simulink model "dfl_model"  (R2022b)
settings: Solver=VariableStepAuto  StartTime=0.0  StopTime=15.0  FixedStep=0.05  RelTol=1e-3
InitFcn:
  | port = 19999;
  | InitSim;
values from neighbouring files (symbols this model uses):
  p = [m, g, I_x, I_y, I_z, c0, c1, c2, c3]'    [dfl_params.m]
  state0 = [x0 y0 z0 v_x0 v_y0 v_z0 phi0 th0 psi0 w_x0 w_y0 w_z0]'    [dfl_params.m]
libraries: VrepLib x1, PosLib x1
settings Model: Creator=dorec  LastModifiedBy=dorec
settings DebuggingCC: SignalInfNanChecking=error

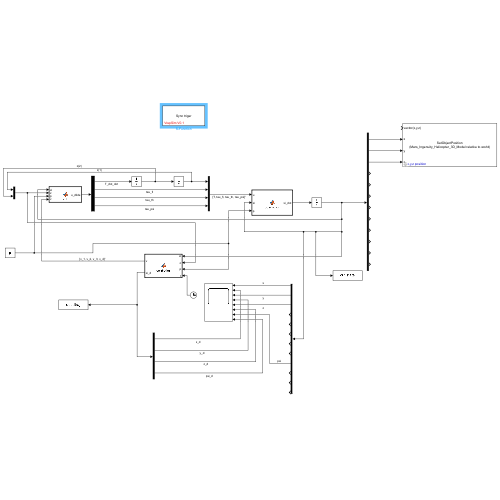
[thumbnail: Simulink's stored preview of the top-level diagram]
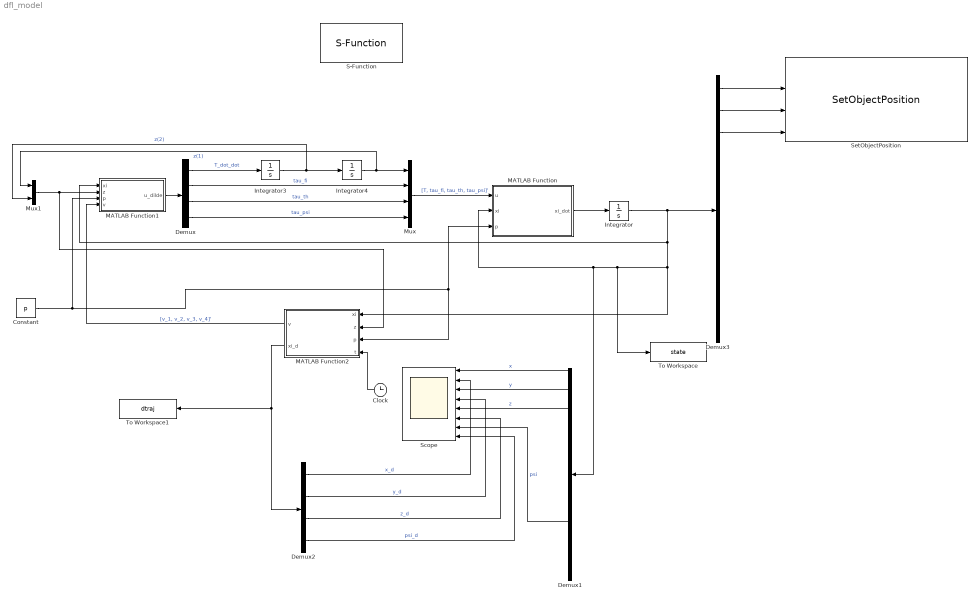
== system dfl_model ==
  Clock : Clock
  Constant : Constant  Value=p
  Demux : Demux
  Demux1 : Demux  Outputs=12
  Demux2 : Demux
  Demux3 : Demux  Outputs=12
  Integrator : Integrator  InitialCondition=state0
  Integrator3 : Integrator
  Integrator4 : Integrator  InitialCondition=1
  MATLAB Function : MATLAB Function  TreatAsAtomicUnit=on
  MATLAB Function1 : MATLAB Function  TreatAsAtomicUnit=on
  MATLAB Function2 : MATLAB Function  TreatAsAtomicUnit=on
  Mux : Mux
  Mux1 : Mux  Inputs=2
  S-Function : VrepLib/S-Function  SFunctionModules=''
      settings: SourceProductName=VrepLib
  Scope : Scope  NumInputPorts=8
  SetObjectPosition : PosLib/SetObjectPosition  object_name='Mars_Ingenuity_Helicopter_3D_Model'  relative_object_name='world'  isUseVector=off
  To Workspace : ToWorkspace  VariableName=state  SaveFormat=Timeseries  SampleTime=-1
  To Workspace1 : ToWorkspace  VariableName=dtraj  SaveFormat=Timeseries  SampleTime=-1
  wires:
  MATLAB Function/1(xi_dot) -> Integrator/1
  Integrator/1 -> MATLAB Function1/1(xi), To Workspace/1, Demux1/1, MATLAB Function/2(xi), MATLAB Function2/1(xi), Demux3/1
  Mux/1 -> MATLAB Function/1(u)  "[T, tau_fi, tau_th, tau_psi]'"
  MATLAB Function1/1(u_dilde) -> Demux/1
  Demux/1 -> Integrator3/1  "T_dot_dot"
  MATLAB Function2/1(v) -> MATLAB Function1/4(v)  "[v_1, v_2, v_3, v_4]'"
  Demux/3 -> Mux/3  "tau_th"
  Demux/2 -> Mux/2  "tau_fi"
  Mux1/1 -> MATLAB Function2/2(z), MATLAB Function1/2(z)
  Constant/1 -> MATLAB Function1/3(p), MATLAB Function/3(p), MATLAB Function2/3(p)
  Clock/1 -> MATLAB Function2/4(t)
  Integrator3/1 -> Mux1/2, Integrator4/1  "z(2)"
  Integrator4/1 -> Mux1/1, Mux/1  "z(1)"
  Demux/4 -> Mux/4  "tau_psi"
  Demux1/1 -> Scope/1  "x"
  Demux1/2 -> Scope/3  "y"
  Demux1/3 -> Scope/5  "z"
  MATLAB Function2/2(xi_d) -> To Workspace1/1, Demux2/1
  Demux2/1 -> Scope/2  "x_d"
  Demux2/2 -> Scope/4  "y_d"
  Demux2/3 -> Scope/6  "z_d"
  Demux2/4 -> Scope/8  "psi_d"
  Demux1/9 -> Scope/7  "psi"
  Demux3/1 -> SetObjectPosition/2
  Demux3/2 -> SetObjectPosition/3
  Demux3/3 -> SetObjectPosition/4

== matlab function dfl_model/MATLAB Function1 ==
  data: xi input size=12; z input size=2; p input size=9; u_dilde output size=4; v input size=4
function u_dilde = dfl(xi, z, p, v)

% x = xi(1);
% y = xi(2);
% z = xi(3);
% v_x = xi(4);
% v_y = xi(5);
% v_z = xi(6);
fi = xi(7);
th = xi(8);
psi = xi(9);
w_x = xi(10);
w_y = xi(11);
w_z = xi(12);

m = p(1);
% g = p(2);
I_x = p(3);
I_y = p(4);
I_z = p(5);

T = z(1);
T_dot = z(2);

J_1 = [-(m*(sin(fi)*sin(psi) + cos(fi)*cos(psi)*sin(th)))/(2*cos(fi)^2*cos(psi)^2 - 2*cos(psi)^2 + 2*cos(psi)^2*cos(th)^2 - 2*cos(fi)^2*cos(psi)^2*cos(th)^2 + 2*cos(fi)*cos(psi)*sin(fi)*sin(psi)*sin(th) + 1), ...
    -(m*(cos(psi)*sin(fi) - 2*cos(psi)*cos(th)^2*sin(fi) + cos(fi)*sin(psi)*sin(th)))/(2*cos(fi)^2*cos(psi)^2 - 2*cos(psi)^2 + 2*cos(psi)^2*cos(th)^2 - 2*cos(fi)^2*cos(psi)^2*cos(th)^2 + 2*cos(fi)*cos(psi)*sin(fi)*sin(psi)*sin(th) + 1), ...
    -(m*cos(th)*(cos(fi) + 2*cos(psi)*sin(fi)*sin(psi)*sin(th)))/(2*cos(fi)^2*cos(psi)^2 - 2*cos(psi)^2 + 2*cos(psi)^2*cos(th)^2 - 2*cos(fi)^2*cos(psi)^2*cos(th)^2 + 2*cos(fi)*cos(psi)*sin(fi)*sin(psi)*sin(th) + 1), ...
    (2*T*cos(psi)*(cos(th)^2 - 1)*(sin(psi) - cos(fi)^2*sin(psi) + cos(fi)*cos(psi)*sin(fi)*sin(th)))/(2*cos(fi)^2*cos(psi)^2 - 2*cos(psi)^2 + 2*cos(psi)^2*cos(th)^2 - 2*cos(fi)^2*cos(psi)^2*cos(th)^2 + 2*cos(fi)*cos(psi)*sin(fi)*sin(psi)*sin(th) + 1)];
J_2 = [-(I_x*m*(cos(fi)*sin(psi) - cos(psi)*sin(fi)*sin(th)))/(T*(2*cos(fi)^2*cos(psi)^2 - 2*cos(psi)^2 + 2*cos(psi)^2*cos(th)^2 - 2*cos(fi)^2*cos(psi)^2*cos(th)^2 + 2*cos(fi)*cos(psi)*sin(fi)*sin(psi)*sin(th) + 1)), ...
    (I_x*m*(cos(fi)*cos(psi) + sin(fi)*sin(psi)*sin(th)))/(T*(2*cos(fi)^2*cos(psi)^2 - 2*cos(psi)^2 + 2*cos(psi)^2*cos(th)^2 - 2*cos(fi)^2*cos(psi)^2*cos(th)^2 + 2*cos(fi)*cos(psi)*sin(fi)*sin(psi)*sin(th) + 1)), ...
    (I_x*m*cos(th)*sin(fi))/(T*(2*cos(fi)^2*cos(psi)^2 - 2*cos(psi)^2 + 2*cos(psi)^2*cos(th)^2 - 2*cos(fi)^2*cos(psi)^2*cos(th)^2 + 2*cos(fi)*cos(psi)*sin(fi)*sin(psi)*sin(th) + 1)), ...
    (I_x*sin(th))/(2*cos(fi)^2*cos(psi)^2 - 2*cos(psi)^2 + 2*cos(psi)^2*cos(th)^2 - 2*cos(fi)^2*cos(psi)^2*cos(th)^2 + 2*cos(fi)*cos(psi)*sin(fi)*sin(psi)*sin(th) + 1)];
J_3 = [-(I_y*m*cos(psi)*cos(th))/(T*cos(fi)*(2*cos(fi)^2*cos(psi)^2 - 2*cos(psi)^2 + 2*cos(psi)^2*cos(th)^2 - 2*cos(fi)^2*cos(psi)^2*cos(th)^2 + 2*cos(fi)*cos(psi)*sin(fi)*sin(psi)*sin(th) + 1)), ...
    -(I_y*m*cos(th)*(sin(psi) + 2*cos(fi)*cos(psi)*sin(fi)*sin(th)))/(T*cos(fi)*(2*cos(fi)^2*cos(psi)^2 - 2*cos(psi)^2 + 2*cos(psi)^2*cos(th)^2 - 2*cos(fi)^2*cos(psi)^2*cos(th)^2 + 2*cos(fi)*cos(psi)*sin(fi)*sin(psi)*sin(th) + 1)), ...
    (I_y*m*(sin(th) - 2*cos(psi)^2*sin(th) + 2*cos(fi)^2*cos(psi)^2*sin(th) + 2*cos(fi)*cos(psi)*sin(fi)*sin(psi) - 2*cos(fi)*cos(psi)*cos(th)^2*sin(fi)*sin(psi)))/(T*cos(fi)*(2*cos(fi)^2*cos(psi)^2 - 2*cos(psi)^2 + 2*cos(psi)^2*cos(th)^2 - 2*cos(fi)^2*cos(psi)^2*cos(th)^2 + 2*cos(fi)*cos(psi)*sin(fi)*sin(psi)*sin(th) + 1)), ...
    -(I_y*cos(th)*(sin(fi) + 2*cos(fi)^2*cos(psi)^2*sin(fi) - 2*cos(fi)^3*cos(psi)*sin(psi)*sin(th) + 2*cos(fi)*cos(psi)*sin(psi)*sin(th) - 2*cos(fi)^2*cos(psi)^2*cos(th)^2*sin(fi)))/(cos(fi)*(2*cos(fi)^2*cos(psi)^2 - 2*cos(psi)^2 + 2*cos(psi)^2*cos(th)^2 - 2*cos(fi)^2*cos(psi)^2*cos(th)^2 + 2*cos(fi)*cos(psi)*sin(fi)*sin(psi)*sin(th) + 1))];
J_4 = [0, 0, 0, I_z];

%J_inv = [J_1; J_2; J_3; J_4];

l_1 = -(-cos(psi)*sin(th)*cos(fi)*(w_z^2) - 2*sin(psi)*cos(th)*cos(fi)*w_y*w_z + 2*sin(psi)*sin(th)*sin(fi)*w_x*w_z - cos(psi)*sin(th)*cos(fi)*(w_y^2) - ...
      2*cos(psi)*cos(th)*sin(fi)*w_y*w_x - cos(psi)*sin(th)*cos(fi)*(w_x^2) - sin(psi)*sin(fi)*(w_z^2) + 2*cos(psi)*cos(fi)*w_z*w_x - ...
      sin(psi)*sin(fi)*(w_x^2))*(T/m) + 2*(-sin(psi)*sin(th)*cos(fi)*w_z + cos(psi)*cos(th)*cos(fi)*w_y - ...
      cos(psi)*sin(th)*sin(fi)*w_x + cos(psi)*sin(fi)*w_z + sin(psi)*cos(fi)*w_x)*(T_dot/m);
l_2 = -(-sin(psi)*sin(th)*cos(fi)*(w_z^2) + 2*cos(psi)*cos(th)*cos(fi)*w_z*w_y - 2*cos(psi)*sin(th)*sin(fi)*w_z*w_x -sin(psi)*sin(th)*cos(fi)*(w_y^2) - ...
      2*sin(psi)*cos(th)*sin(fi)*w_y*w_x - sin(psi)*sin(th)*cos(fi)*(w_x^2) + sin(fi)*cos(psi)*(w_x^2) + 2*cos(fi)*sin(psi)*w_x*w_z + ...
      sin(fi)*cos(psi)*(w_z^2))*(T/m) - 2*(cos(psi)*sin(th)*cos(fi)*w_z + sin(psi)*cos(th)*cos(fi)*w_y - ...
      sin(psi)*sin(th)*sin(fi)*w_x - cos(fi)*cos(psi)*w_x + sin(fi)*sin(psi)*w_z)*(T_dot/m);
l_3 = cos(th)*cos(fi)*(w_y^2)*(T/m) - 2*sin(th)*sin(fi)*w_x*w_y*(T/m) + 2*sin(th)*cos(fi)*w_y*(T_dot/m) + cos(th)*cos(fi)*(w_x^2)*(T/m) + 2*cos(th)*sin(fi)*w_x*(T_dot/m);
l_4 = 0;

l = [l_1; l_2; l_3; l_4];

T_dot_dot = J_1*(-l + v);
tau_fi = J_2*(-l + v);
tau_th = J_3*(-l + v);
tau_psi = J_4*(-l + v);

u_dilde = [T_dot_dot, tau_fi, tau_th, tau_psi]';

== matlab function dfl_model/MATLAB Function ==
  data: u input size=4; xi_dot output size=12; xi input size=12; p input size=9
function xi_dot = quadrotor(u, xi, p)

T = u(1);
tau_fi = u(2);
tau_th = u(3);
tau_psi = u(4);

% x = xi(1);
% y = xi(2);
% z = xi(3);
v_x = xi(4);
v_y = xi(5);
v_z = xi(6);
fi = xi(7);
th = xi(8);
psi = xi(9);
w_x = xi(10);
w_y = xi(11);
w_z = xi(12);

m = p(1);
g = p(2);
I_x = p(3);
I_y = p(4);
I_z = p(5);

x_dot = v_x;
v_x_dot = -(cos(psi)*sin(th)*cos(fi) + sin(psi)*sin(fi))*(T/m);
y_dot = v_y;
v_y_dot = -(sin(psi)*sin(th)*cos(fi) - sin(fi)*cos(psi))*(T/m);
z_dot = v_z;
v_z_dot = -cos(th)*cos(fi)*(T/m) + g;
fi_dot = w_x;
w_x_dot = tau_fi/I_x;
th_dot = w_y;
w_y_dot = tau_th/I_y;
psi_dot = w_z;
w_z_dot = tau_psi/I_z;

xi_dot = [x_dot, y_dot, z_dot, v_x_dot, v_y_dot, v_z_dot, fi_dot, th_dot, psi_dot, w_x_dot, w_y_dot, w_z_dot]';

== matlab function dfl_model/MATLAB Function2 ==
  data: xi input size=12; v output size=4; z input size=2; p input size=9; t input; xi_d output
function [v,xi_d] = controller(xi, z, p, t)

eta_1 = xi(1); % x
eta_2 = xi(2); % y
eta_3 = xi(3); % z
v_x = xi(4);
v_y = xi(5);
v_z = xi(6);
fi = xi(7);
th = xi(8);
eta_4 = xi(9); % psi
w_x = xi(10);
w_y = xi(11);
w_z = xi(12);

T = z(1);
T_dot = z(2);

m = p(1);
g = p(2);
c0 = p(6);
c1 = p(7);
c2 = p(8);
c3 = p(9);

%% Spiral
x_d = cos(t);
y_d = sin(t);
z_d = 1 + (t/10);
psi_d = pi/2;

%% Parabolic
% x_d = t;
% y_d = t;
% z_d = -(1/15)*t^2 + t;
% psi_d = pi/2;

xi_d = [x_d, y_d, z_d, psi_d]';

eta_1_d = xi_d(1);
eta_2_d = xi_d(2);
eta_3_d = xi_d(3);
eta_4_d = xi_d(4);

%% Spiral derivatives
eta_1_d_dot1 = -sin(t);
eta_1_d_dot2 = -cos(t);
eta_1_d_dot3 = sin(t);
eta_1_d_dot4 = cos(t);
eta_2_d_dot1 = cos(t);
eta_2_d_dot2 = -sin(t);
eta_2_d_dot3 = -cos(t);
eta_2_d_dot4 = sin(t);
eta_3_d_dot1 = 1/10;
eta_3_d_dot2 = 0;
eta_3_d_dot3 = 0;
eta_3_d_dot4 = 0;
eta_4_d_dot1 = 0;
eta_4_d_dot2 = 0;

%% Parabolic derivatives
% eta_1_d_dot1 = 1;
% eta_1_d_dot2 = 0;
% eta_1_d_dot3 = 0;
% eta_1_d_dot4 = 0;
% eta_2_d_dot1 = 1;
% eta_2_d_dot2 = 0;
% eta_2_d_dot3 = 0;
% eta_2_d_dot4 = 0;
% eta_3_d_dot1 = -(2/15)*t + 1;
% eta_3_d_dot2 = -(2/15);
% eta_3_d_dot3 = 0;
% eta_3_d_dot4 = 0;
% eta_4_d_dot1 = 0;
% eta_4_d_dot2 = 0;

eta_1_dot1 = v_x;
eta_1_dot2 = -(cos(eta_4)*sin(th)*cos(fi) + sin(eta_4)*sin(fi))*(T/m);
eta_1_dot3 = -(-sin(eta_4)*sin(th)*cos(fi)*w_z + cos(eta_4)*cos(th)*cos(fi)*w_y - cos(eta_4)*sin(th)*sin(fi)*w_x + ...
             cos(eta_4)*sin(fi)*w_z + sin(eta_4)*cos(fi)*w_x)*(T/m) - ...
             (cos(eta_4)*sin(th)*cos(fi) + sin(eta_4)*sin(fi))*(T_dot/m);
eta_2_dot1 = v_y;
eta_2_dot2 = -(sin(eta_4)*sin(th)*cos(fi) - sin(fi)*cos(eta_4))*(T/m);
eta_2_dot3 = -(cos(eta_4)*sin(th)*cos(fi)*w_z + sin(eta_4)*cos(th)*cos(fi)*w_y - sin(eta_4)*sin(th)*sin(fi)*w_x - ...
             cos(fi)*cos(eta_4)*w_x + sin(fi)*sin(eta_4)*w_z)*(T/m) - ...
             (sin(eta_4)*sin(th)*cos(fi) - sin(fi)*cos(eta_4))*(T_dot/m);
eta_3_dot1 = v_z;
eta_3_dot2 = -cos(th)*cos(fi)*(T/m) + g;
eta_3_dot3 = (sin(th)*cos(fi)*w_y + cos(th)*sin(fi)*w_x)*(T/m) - cos(th)*cos(fi)*(T_dot/m);
eta_4_dot1 = xi(12);

e10 = eta_1_d - eta_1;
e11 = eta_1_d_dot1 - eta_1_dot1;
e12 = eta_1_d_dot2 - eta_1_dot2;
e13 = eta_1_d_dot3 - eta_1_dot3;
e20 = eta_2_d - eta_2;
e21 = eta_2_d_dot1 - eta_2_dot1;
e22 = eta_2_d_dot2 - eta_2_dot2;
e23 = eta_2_d_dot3 - eta_2_dot3;
e30 = eta_3_d - eta_3;
e31 = eta_3_d_dot1 - eta_3_dot1;
e32 = eta_3_d_dot2 - eta_3_dot2;
e33 = eta_3_d_dot3 - eta_3_dot3;
e40 = eta_4_d - eta_4;
e41 = eta_4_d_dot1 - eta_4_dot1;

v_1 = c0*e10 + c1*e11 + c2*e12 + c3*e13 + eta_1_d_dot4;
v_2 = c0*e20 + c1*e21 + c2*e22 + c3*e23 + eta_2_d_dot4;
v_3 = c0*e30 + c1*e31 + c2*e32 + c3*e33 + eta_3_d_dot4;
v_4 = c0*e40 + c1*e41 + eta_4_d_dot2;

v = [v_1, v_2, v_3, v_4]';
